simulink model "pid_controller"  (R2016a)
settings: Solver=VariableStepAuto  StartTime=0.0  StopTime=20  RelTol=1e-3
values from neighbouring files (symbols this model uses):
  B = ((Kt/K)-Ke*Kt)/R    [SkinnerJ_FinalProject.m]
  J = 0.1306    [Root_Locus.m]    (also in SkinnerJ_FinalProject.m = (tau*(R*B + Ke*Kt))/R)
  Kd = 0.5    [Final_Project_Auger_motor.m]    (also in SkinnerJ_FinalProject.m = 0)
  Ki = 37    [Final_Project_Auger_motor.m]    (also in SkinnerJ_FinalProject.m = 0.05)
  Kp = .5    (= 0.5)    [Final_Project_Auger_motor.m]    (also in SkinnerJ_FinalProject.m = 0.4)
  Kt = Td*R/6    [SkinnerJ_FinalProject.m]
  R = 4    [Root_Locus.m]    (also in SkinnerJ_FinalProject.m)
  Target = 120    [SkinnerJ_FinalProject.m]
libraries: simulink x1
settings Model: Creator=jds10  LastModifiedBy=zf1005

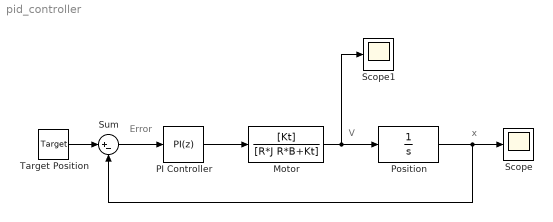
== system pid_controller ==
  note: x
  note: V
  note: Error
  Motor : TransferFcn  Numerator=[Kt]  Denominator=[R*J R*B+Kt]
  PI Controller : simulink/Continuous/PID Controller  Controller=PI  TimeDomain=Discrete-time  SampleTime=0.01  IntegratorMethod=Backward Euler  FilterMethod=Backward Euler  Form=Parallel  UseFilter=on  ControllerParametersSource=internal  P=Kp  I=Ki  D=Kd  N=10000  InitialConditionSource=internal  InitialConditionForIntegrator=0  InitialConditionForFilter=0  ExternalReset=none  LimitOutput=off  UpperSaturationLimit=inf  LowerSaturationLimit=-inf  LinearizeAsGain=on  AntiWindupMode=none  Kb=1  TrackingMode=off  Kt=1  PParamMin=[]  PParamMax=[]  IParamMin=[]  IParamMax=[]  DParamMin=[]  DParamMax=[]  NParamMin=[]  NParamMax=[]  KbParamMin=[]  KbParamMax=[]  KtParamMin=[]  KtParamMax=[]  POutMin=[]  POutMax=[]  IOutMin=[]  IOutMax=[]  DOutMin=[]  DOutMax=[]  NOutMin=[]  NOutMax=[]  KbOutMin=[]  KbOutMax=[]  KtOutMin=[]  KtOutMax=[]  IntegratorOutMin=[]  IntegratorOutMax=[]  FilterOutMin=[]  FilterOutMax=[]  SumOutMin=[]  SumOutMax=[]  SumI1OutMin=[]  SumI1OutMax=[]  SumI2OutMin=[]  SumI2OutMax=[]  SumI3OutMin=[]  SumI3OutMax=[]  SumDOutMin=[]  SumDOutMax=[]  SaturationOutMin=[]  SaturationOutMax=[]  IntegratorContinuousStateAttributes=''  IntegratorStateMustResolveToSignalObject=off  IntegratorRTWStateStorageClass=Auto  FilterContinuousStateAttributes=''  FilterStateMustResolveToSignalObject=off  FilterRTWStateStorageClass=Auto  DifferentiatorICPrevScaledInput=0  DifferentiatorOutMin=[]  DifferentiatorOutMax=[]
  Position : TransferFcn  Denominator=[1 0]
  Scope : Scope
  Scope1 : Scope
  Sum : Sum  Inputs=|+-
  Target Position : Constant  Value=Target
  wires:
  Target Position/1 -> Sum/1
  Sum/1 -> PI Controller/1
  PI Controller/1 -> Motor/1
  Motor/1 -> Scope1/1, Position/1
  Position/1 -> Sum/2, Scope/1
